simulink model "SimMain"  (R2019a)
settings: Solver=VariableStepAuto  StartTime=0.0  StopTime=inf  MaxStep=1  RelTol=1e-3
InitFcn:
  | Model;
libraries: roblocks x2
settings Model: Creator=Administrator  LastModifiedBy=Cybaster
settings DataIOCC: ReturnWorkspaceOutputs=off
settings DebuggingCC: ArithmeticOperatorsInVariantConditions=warning

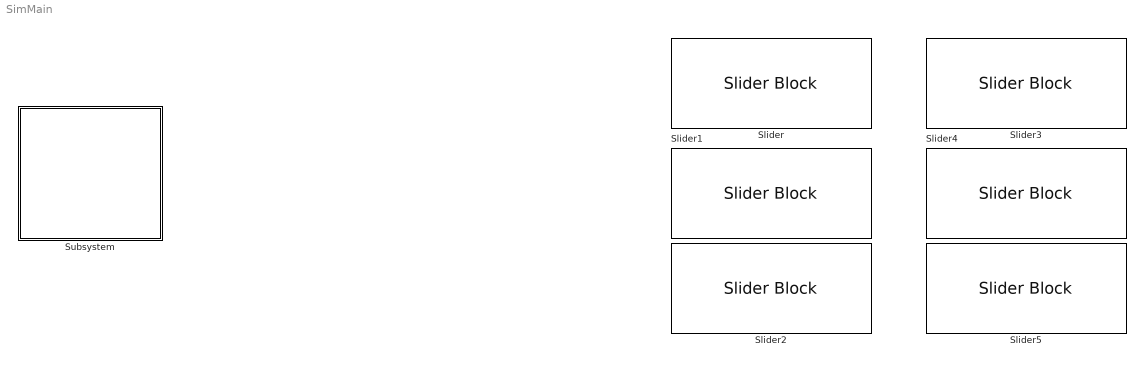
== system SimMain ==
  Slider{,1..5} (6 alike) : SliderBlock  ScaleMin=-1  ScaleMax=1
  Subsystem : Subsystem

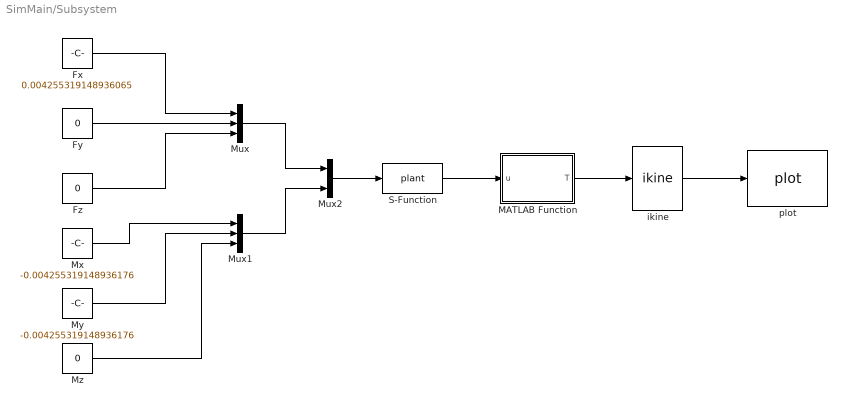
== system SimMain/Subsystem ==
  Fx : Constant  Value=0.004255319148936065
  Fy : Constant  Value=0
  Fz : Constant  Value=0
  MATLAB Function : MATLAB Function  TreatAsAtomicUnit=on
  Mux : Mux  Inputs=3
  Mux1 : Mux  Inputs=3
  Mux2 : Mux  Inputs=2
  Mx : Constant  Value=-0.004255319148936176
  My : Constant  Value=-0.004255319148936176
  Mz : Constant  Value=0
  S-Function : S-Function  FunctionName=plant  SFunctionDeploymentMode=off  EnableBusSupport=off
  ikine : roblocks/Arm/ikine  robot=robot  q0=[0, 0, 0, 0, -2*pi/3, 0]  M=[1 1 1 1 1 1]  pinv=off  options={}
  plot : roblocks/Arm/plot  robot=robot  fps=5  holdplot=off
  wires:
  S-Function/1 -> MATLAB Function/1(u)
  My/1 -> Mux1/2
  Mux/1 -> Mux2/1
  Mz/1 -> Mux1/3
  Fx/1 -> Mux/1
  Fy/1 -> Mux/2
  Fz/1 -> Mux/3
  Mux2/1 -> S-Function/1
  ikine/1 -> plot/1
  Mx/1 -> Mux1/1
  Mux1/1 -> Mux2/2
  MATLAB Function/1(T) -> ikine/1

== matlab function SimMain/Subsystem/MATLAB Function ==
  data: u input; T output
function T = fcn(u)
x0 = 0.5; y0 = 0; z0 = 0.8;
roll0 = 0; pitch0 = 0; yaw0 = pi;
p0 = [x0; y0; z0];
R0 = rotX(yaw0) * rotY(pitch0) * rotZ(roll0);
T0 = eye(4);
T0(1:3, 1:3) = R0;
T0(1:3, 4) = p0;

Xe = u(1); Ye = u(2); Ze = u(3);
phi = u(7); theta = u(8); psi = u(9);
pe = [Xe; Ye; Ze];
Re = xyz2R(phi, theta, psi);

T = T0;
T(1:3, 4) = T(1:3, 4) + pe;
T(1:3, 1:3) = Re * R0;
